simulink model "Classical_PTC_simo"  (R2016a)
settings: Solver=FixedStepAuto  StartTime=0.0  StopTime=3.8  FixedStep=1e-6  MaxStep=4e-6  RelTol=1e-6
values from neighbouring files (symbols this model uses):
  alpbet = [2/3, -1/3, -1/3; 0, sqrt(3)/3, -sqrt(3)/3 ]    [params_for_simo_Nisan21.m]
  kr = Lm/Lr    (= 0.98)    [params_for_simo_Nisan21.m]
  Lambda = 50    [params_for_simo_Nisan21.m]
  NTlimit = -3    [params_for_simo_Nisan21.m]
  OCLimit = 10    [params_for_simo_Nisan21.m]
  PhisRef = 0.3    [params_for_simo_Nisan21.m]
  PP = 1    [params_for_simo_Nisan21.m]
  PTlimit = 3    [params_for_simo_Nisan21.m]
  Req = Rs+kr*kr*Rr    (= 5.27724)    [params_for_simo_Nisan21.m]
  Rs = 2.3    [params_for_simo_Nisan21.m]
  taur = Lr/Rr    (= 0.0322580645161)    [params_for_simo_Nisan21.m]
  taus = Lstr/Req    (= 0.00112937823559)    [params_for_simo_Nisan21.m]
  Tmpc = T    (= 2.5e-05)    [params_for_simo_Nisan21.m]
undefined symbols (not defined in the file or in its folder): DiscIntNeverNeededParam
libraries: powerlib x7, simulink x2
settings Model: NumberOfSteps=30  Creator=pc  LastModifiedBy=silker
settings SolverCC: AlgebraicLoopSolver=LineSearch

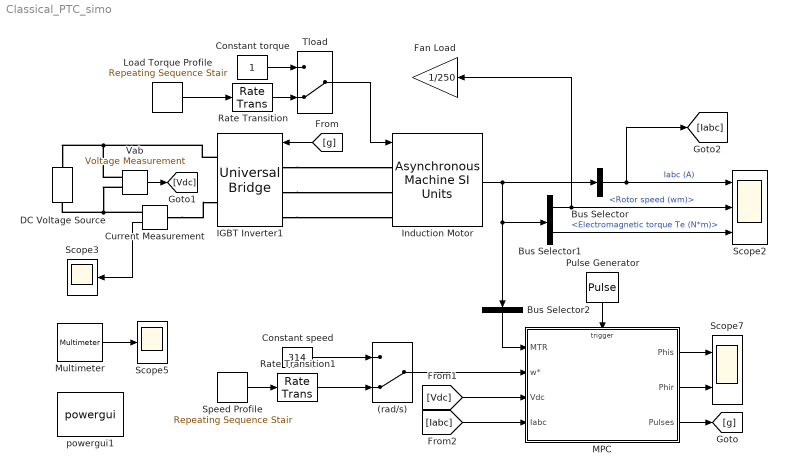
== system Classical_PTC_simo ==
  (rad/s) : ManualSwitch  CurrentSetting=0
  Bus Selector : BusSelector  OutputSignals=Stator measurements.Stator current is_a (A),Stator measurements.Stator current is_b (A),Stator measurements.Stator current is_c (A)  OutputAsBus=on
  Bus Selector1 : BusSelector  OutputSignals=Mechanical.Rotor speed (wm),Mechanical.Electromagnetic torque Te (N*m)
  Bus Selector2 : BusSelector  OutputSignals=Stator measurements.Stator flux phis_q (V s),Stator measurements.Stator flux phis_d (V s),Rotor measurements.Rotor flux phir_q (V s),Rotor measurements.Rotor flux phir_d (V s),Mechanical.Rotor speed (wm)  OutputAsBus=on
  Constant speed : Constant  Value=314
  Constant torque : Constant
  Current Measurement : powerlib/Measurements/Current Measurement  PhasorSimulation=off  OutputType=Complex  PSBequivalent=0
  DC Voltage Source : powerlib/Electrical Sources/DC Voltage Source  Amplitude=350  Measurements=None
  Fan Load : Gain  Gain=1/250
  IGBT Inverter1 : powerlib/Power Electronics/Universal Bridge  Arms=3  SnubberResistance=1e6  SnubberCapacitance=1e-9  Device=IGBT / Diodes  Ron=1e-3  Lon=0  ForwardVoltages="[  0.8  0.8  ]"  ForwardVoltage=.8  GTOparameters=[ 1e-6 , 1e-6 ]  IGBTparameters=[ 1e-6 , 2e-6 ]  Measurements=All voltages and currents  Measurements_2=None  converterType=Rectifier
  Induction Motor : powerlib/Machines/Asynchronous Machine SI Units  RotorType=Squirrel-cage  PresetModel=No  MechanicalLoad=Torque Tm  ShowDetailedParameters=on  ReferenceFrame=Stationary  Units=SI  MeasurementBus=off  NominalParameters=[ 1500, 380, 50 ]  Stator=[ 2.3 4e-3 ]  Rotor="[3.1  2e-3 ]"  Cage1=[ 0.022 0.226/377]  Cage2=[ 0.022 0.226/377]  Lm=98e-3  Mechanical="[0.003  0.0005 1 ]"  PolePairs=2  InitialConditions="[ 1, 0 ,  0 , 0 , 0 , 0 , 0 , 0 ]"  SimulateSaturation=off  Saturation=[0 0;0 0]  LoadFlowParameters=0  TsPowergui=0  TsBlock=-1  IterativeModel=Trapezoidal non iterative  IterativeDiscreteModel=Trapezoidal non iterative  Pmec=0
  Load Torque Profile : simulink/Sources/Repeating Sequence Stair  OutValues="[0.7 0.7 0.7 0.7 0.7 0.7 0.7 0.7 0.7 0.7 1.35 1.35 1.35 1.35 1.35 1.35 1.35 1.35 1.35  -0.3 -0.3 -0.3 -0.3 -0.3 -0.3 -0.3 -0.3 -0.3 -0.3 -1.35 -1.35 -1.35 -1.35 -1.35 -0.7 -0.7 -0.7 -0.7 ]"  tsamp=0.1  OutMin=[]  OutMax=[]  OutDataTypeStr=double  OutputDataTypeScalingMode=double  OutDataType=fixdt(0,8)  ConRadixGroup=Best Precision: Vector-wise  OutScaling=2^-12
  MPC : Subsystem  TreatAsAtomicUnit=on
  Multimeter : powerlib/Measurements/Multimeter  PhasorSimulation=off  OutputType=Complex  sel=11  L=16  Gain=1  yselected={'Isw1: IGBT Inverter1'};  PSBOutputType=1  PSBequivalent=0  AxesSetting=[0,0.1,-100,100]  Display=0  SavedBlockNames=-11
  Pulse Generator : DiscretePulseGenerator  PulseType=Time based  Period=Tmpc  PulseWidth=40
  Rate Transition : RateTransition  X0=0.7
  Rate Transition1 : RateTransition  X0=300
  Scope2 : Scope  NumInputPorts=3
  Scope3 : Scope
  Scope5 : Scope
  Scope7 : Scope  NumInputPorts=2
  Speed Profile : simulink/Sources/Repeating Sequence Stair  OutValues=[ 300 300 300 300 300 300 300 150 150 150 150 150 150 300 300 300 300 300 300 -300 -300 -300 -300 -300 -300 -300 -300 -300 -300 -300 -300 -150 -150 -150 -150 -150 -150 -150]  tsamp=0.1  OutMin=[]  OutMax=[]  OutDataTypeStr=double  OutputDataTypeScalingMode=double  OutDataType=fixdt(0,8)  ConRadixGroup=Best Precision: Vector-wise  OutScaling=2^-12
  Tload : ManualSwitch  CurrentSetting=0
  Vab : powerlib/Measurements/Voltage Measurement  Tag=PoWeRsYsTeMmEaSuReMeNt  PhasorSimulation=off  OutputType=Magnitude  PSBequivalent=0
  powergui1 : powerlib/powergui  Priority=1  SimulationMode=Discrete  SolverType=Tustin/Backward Euler (TBE)  SampleTime=1e-6  frequency=60  SPID=off  DisableSnubberDevices=off  DisableRonSwitches=off  DisableVfSwitches=off  SwTol=0  DisplayEquations=off  Interpol=off  ExternalGateDelay=off  methode=off  Ts=10  FunctionMessages=off  echomessages=off  HookPort=off  EnableUseOfTLC=off  x0status=blocks  frequencyindice=0  Pbase=100e6  ErrMax=1e-4  Iterations=50  UnitsV=kV  UnitsW=MW  buscounter=0  RestoreLinks=warning  ResistiveCurrentMeasurement=off  Frange=[0:2:500]  Ylog=off  Xlog=on  ShowGrid=off  save=off  variable=ZData  structure=classical_cur  ZoomFFT=off  StartTime=0.305  cycles=20  DisplayStyle=1  fundamental=33  FreqAxis=off  MaxFrequency=10000  frequencyindicesteady=1  RmsSteady=1  display=off
  wires:
  Pulse Generator/1 -> MPC/Trigger
  Load Torque Profile/1 -> Rate Transition/1
  Constant torque/1 -> Tload/1
  Induction Motor/1 -> Bus Selector/1, Bus Selector2/1, Bus Selector1/1
  Bus Selector2/1 -> MPC/1(MTR)
  MPC/3(Pulses) -> [g]
  [g] -> IGBT Inverter1/1
  Constant speed/1 -> (rad/s)/1
  Rate Transition1/1 -> (rad/s)/2
  Vab/1 -> [Vdc]
  [Vdc] -> MPC/3(Vdc)
  Rate Transition/1 -> Tload/2
  Current Measurement/1 -> Scope3/1
  (rad/s)/1 -> MPC/2(w*)
  Bus Selector1/1 -> Scope2/2, Fan Load/1  "<Rotor speed (wm)>"
  Bus Selector1/2 -> Scope2/3  "<Electromagnetic torque Te (N*m)>"
  [Iabc] -> MPC/4(Iabc)
  Bus Selector/1 -> Scope2/1, [Iabc]  "Iabc (A)"
  Multimeter/1 -> Scope5/1
  MPC/1(Phis) -> Scope7/1
  MPC/2(Phir) -> Scope7/2
  Speed Profile/1 -> Rate Transition1/1
  Tload/1 -> Induction Motor/1
  connections:
  Vab/LConn2 -- DC Voltage Source/LConn1 -- Current Measurement/RConn1
  IGBT Inverter1/RConn1 -- Vab/LConn1 -- DC Voltage Source/RConn1
  IGBT Inverter1/LConn1 -- Induction Motor/LConn1
  IGBT Inverter1/LConn2 -- Induction Motor/LConn2
  IGBT Inverter1/LConn3 -- Induction Motor/LConn3
  Current Measurement/LConn1 -- IGBT Inverter1/RConn2

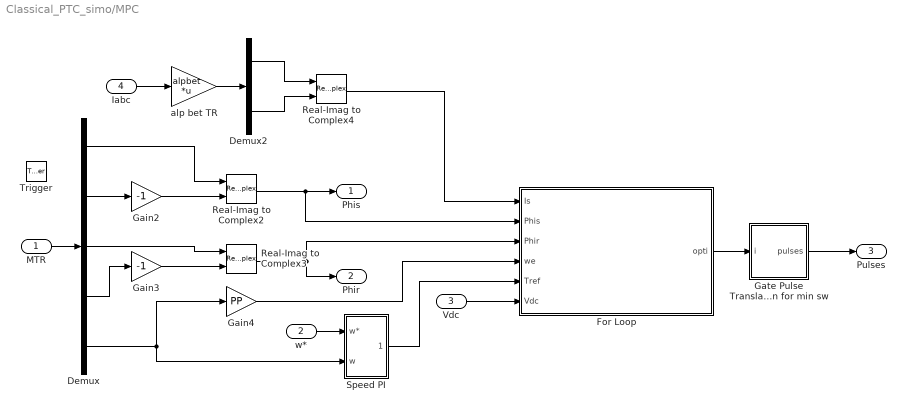
== system Classical_PTC_simo/MPC ==
  MTR : Inport
  w* : Inport  Port=2
  Vdc : Inport  Port=3
  Iabc : Inport  Port=4
  Trigger : TriggerPort  VariantControl=Variant
  Demux : Demux  Outputs=5
  Demux2 : Demux  Outputs=2
  For Loop : Subsystem  TreatAsAtomicUnit=on
  Gain2 : Gain  Gain=-1
  Gain3 : Gain  Gain=-1
  Gain4 : Gain  Gain=PP
  Gate Pulse Translation for min sw : Subsystem
  Real-Imag to Complex2 : RealImagToComplex
  Real-Imag to Complex3 : RealImagToComplex
  Real-Imag to Complex4 : RealImagToComplex
  Speed PI : Subsystem
  alp bet TR : Gain  Gain=alpbet  Multiplication=Matrix(K*u)
  Phis : Outport
  Phir : Outport  Port=2
  Pulses : Outport  Port=3
  wires:
  MTR/1 -> Demux/1
  Gain3/1 -> Real-Imag to Complex3/2
  Gain2/1 -> Real-Imag to Complex2/2
  Real-Imag to Complex2/1 -> For Loop/2(Phis), Phis/1
  Real-Imag to Complex3/1 -> For Loop/3(Phir), Phir/1
  w*/1 -> Speed PI/1(w*)
  Gain4/1 -> For Loop/4(we)
  Speed PI/1(Te*) -> For Loop/5(Tref)
  Vdc/1 -> For Loop/6(Vdc)
  Gate Pulse Translation for min sw/1(pulses) -> Pulses/1
  For Loop/1(opti) -> Gate Pulse Translation for min sw/1(i)
  Demux/1 -> Real-Imag to Complex2/1
  Demux/2 -> Gain2/1
  Demux/3 -> Real-Imag to Complex3/1
  Demux/4 -> Gain3/1
  Demux/5 -> Gain4/1, Speed PI/2(w)
  Iabc/1 -> alp bet TR/1
  Demux2/2 -> Real-Imag to Complex4/2
  Demux2/1 -> Real-Imag to Complex4/1
  alp bet TR/1 -> Demux2/1
  Real-Imag to Complex4/1 -> For Loop/1(Is)

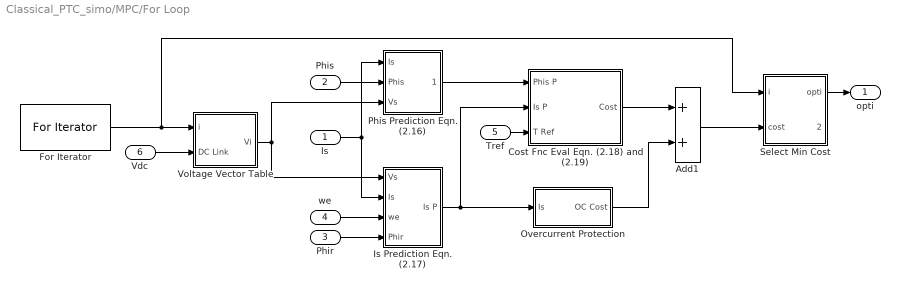
== system Classical_PTC_simo/MPC/For Loop ==
  Is : Inport
  Phis : Inport  Port=2
  Phir : Inport  Port=3
  we : Inport  Port=4
  Tref : Inport  Port=5
  Vdc : Inport  Port=6
  Add1 : Sum
  Cost Fnc Eval Eqn. (2.18) and (2.19) : Subsystem
  For Iterator : ForIterator  IterationLimit=7  IterationVariableDataType=double
  Is Prediction Eqn. (2.17) : Subsystem
  Overcurrent Protection : Subsystem
  Phis Prediction Eqn. (2.16) : Subsystem
  Select Min Cost : Subsystem
  Voltage Vector Table : Subsystem
  opti : Outport
  wires:
  Select Min Cost/1(opti) -> opti/1
  Voltage Vector Table/1(Vi) -> Phis Prediction Eqn. (2.16)/3(Vs), Is Prediction Eqn. (2.17)/1(Vs)
  Phis Prediction Eqn. (2.16)/1(Phis P) -> Cost Fnc Eval Eqn. (2.18) and (2.19)/1(Phis P)
  Is Prediction Eqn. (2.17)/1(Is P) -> Overcurrent Protection/1(Is), Cost Fnc Eval Eqn. (2.18) and (2.19)/2(Is P)
  Cost Fnc Eval Eqn. (2.18) and (2.19)/1(Cost) -> Add1/1
  Overcurrent Protection/1(OC Cost) -> Add1/2
  Is/1 -> Is Prediction Eqn. (2.17)/2(Is), Phis Prediction Eqn. (2.16)/1(Is)
  Phis/1 -> Phis Prediction Eqn. (2.16)/2(Phis)
  Phir/1 -> Is Prediction Eqn. (2.17)/4(Phir)
  we/1 -> Is Prediction Eqn. (2.17)/3(we)
  Vdc/1 -> Voltage Vector Table/2(DC Link)
  Tref/1 -> Cost Fnc Eval Eqn. (2.18) and (2.19)/3(T Ref)
  Add1/1 -> Select Min Cost/2(cost)
  For Iterator/1 -> Select Min Cost/1(i), Voltage Vector Table/1(i)

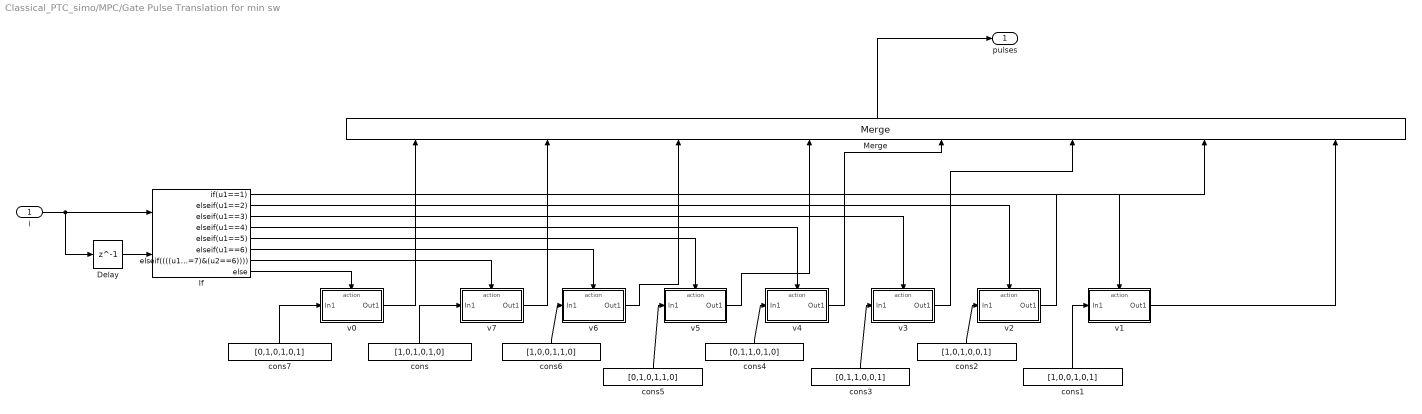
== system Classical_PTC_simo/MPC/Gate Pulse Translation for min sw ==
  i : Inport
  Delay : Delay  DelayLength=1  InitialCondition=0
  If : If  NumInputs=2  IfExpression=u1==1  ElseIfExpressions=u1==2, u1==3, u1==4, u1==5, u1==6,(((u1==7)&(u2==2)) | ((u1==7)&(u2==4)) | ((u1==7)&(u2==6)))
  Merge : Merge  Inputs=8
  cons : Constant  Value=[1,0,1,0,1,0]
  cons1 : Constant  Value=[1,0,0,1,0,1]
  cons2 : Constant  Value=[1,0,1,0,0,1]
  cons3 : Constant  Value=[0,1,1,0,0,1]
  cons4 : Constant  Value=[0,1,1,0,1,0]
  cons5 : Constant  Value=[0,1,0,1,1,0]
  cons6 : Constant  Value=[1,0,0,1,1,0]
  cons7 : Constant  Value=[0,1,0,1,0,1]
  v0 : Subsystem  TreatAsAtomicUnit=on
  v1 : Subsystem  TreatAsAtomicUnit=on
  v2 : Subsystem  TreatAsAtomicUnit=on
  v3 : Subsystem  TreatAsAtomicUnit=on
  v4 : Subsystem  TreatAsAtomicUnit=on
  v5 : Subsystem  TreatAsAtomicUnit=on
  v6 : Subsystem  TreatAsAtomicUnit=on
  v7 : Subsystem  TreatAsAtomicUnit=on
  pulses : Outport
  wires:
  i/1 -> Delay/1, If/1
  If/1 -> v1/Action
  Merge/1 -> pulses/1
  cons/1 -> v7/1(In1)
  If/3 -> v3/Action
  If/2 -> v2/Action
  If/4 -> v4/Action
  If/5 -> v5/Action
  If/7 -> v7/Action
  If/6 -> v6/Action
  cons1/1 -> v1/1(In1)
  cons2/1 -> v2/1(In1)
  cons3/1 -> v3/1(In1)
  cons4/1 -> v4/1(In1)
  cons5/1 -> v5/1(In1)
  cons6/1 -> v6/1(In1)
  Delay/1 -> If/2
  cons7/1 -> v0/1(In1)
  If/8 -> v0/Action
  v0/1(Out1) -> Merge/1
  v7/1(Out1) -> Merge/2
  v6/1(Out1) -> Merge/3
  v5/1(Out1) -> Merge/4
  v4/1(Out1) -> Merge/5
  v3/1(Out1) -> Merge/6
  v2/1(Out1) -> Merge/7
  v1/1(Out1) -> Merge/8

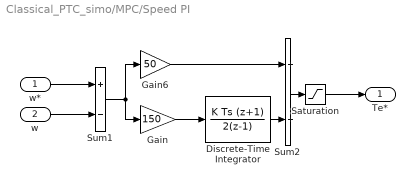
== system Classical_PTC_simo/MPC/Speed PI ==
  w* : Inport
  w : Inport  Port=2
  Discrete-Time Integrator : DiscreteIntegrator  IntegratorMethod=Integration: Trapezoidal  SampleTime=-1  LimitOutput=on  UpperSaturationLimit=90  LowerSaturationLimit=-90  ICPrevOutput=DiscIntNeverNeededParam  ICPrevScaledInput=DiscIntNeverNeededParam
  Gain : Gain  Gain=150  SaturateOnIntegerOverflow=on  OutDataTypeStr=Inherit: Same as input  ParamDataTypeStr=Inherit: Same as input
  Gain6 : Gain  Gain=50  SaturateOnIntegerOverflow=on  OutDataTypeStr=Inherit: Same as input  ParamDataTypeStr=Inherit: Same as input
  Saturation : Saturate  UpperLimit=PTlimit  LowerLimit=NTlimit
  Sum1 : Sum  Inputs=+-  SaturateOnIntegerOverflow=on  InputSameDT=on  OutDataTypeStr=Inherit: Same as first input
  Sum2 : Sum  SaturateOnIntegerOverflow=on  InputSameDT=on  OutDataTypeStr=Inherit: Same as first input
  Te* : Outport  InitialOutput=0
  wires:
  Gain/1 -> Discrete-Time Integrator/1
  Sum1/1 -> Gain/1, Gain6/1
  Gain6/1 -> Sum2/1
  Saturation/1 -> Te*/1
  w*/1 -> Sum1/1
  w/1 -> Sum1/2
  Discrete-Time Integrator/1 -> Sum2/2
  Sum2/1 -> Saturation/1

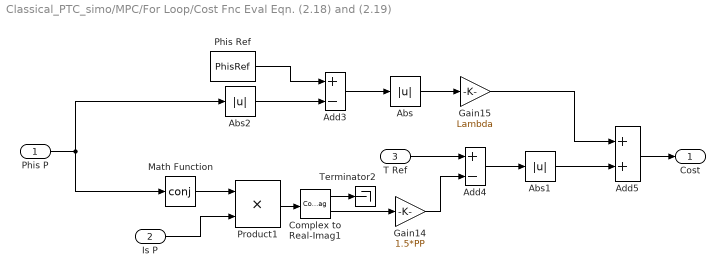
== system Classical_PTC_simo/MPC/For Loop/Cost Fnc Eval Eqn. (2.18) and (2.19) ==
  Phis P : Inport
  Is P : Inport  Port=2
  T Ref : Inport  Port=3
  Abs : Abs
  Abs1 : Abs
  Abs2 : Abs
  Add3 : Sum  Inputs=+-
  Add4 : Sum  Inputs=+-
  Add5 : Sum
  Complex to Real-Imag1 : ComplexToRealImag
  Gain14 : Gain  Gain=1.5*PP
  Gain15 : Gain  Gain=Lambda
  Math Function : Math  Operator=conj  SaturateOnIntegerOverflow=on
  Phis Ref : Constant  Value=PhisRef
  Product1 : Product
  Terminator2 : Terminator
  Cost : Outport
  wires:
  Phis P/1 -> Abs2/1, Math Function/1
  Complex to Real-Imag1/1 -> Terminator2/1
  Is P/1 -> Product1/2
  Product1/1 -> Complex to Real-Imag1/1
  Math Function/1 -> Product1/1
  Add3/1 -> Abs/1
  Gain14/1 -> Add4/2
  Phis Ref/1 -> Add3/1
  T Ref/1 -> Add4/1
  Abs1/1 -> Add5/2
  Add5/1 -> Cost/1
  Add4/1 -> Abs1/1
  Gain15/1 -> Add5/1
  Abs/1 -> Gain15/1
  Complex to Real-Imag1/2 -> Gain14/1
  Abs2/1 -> Add3/2

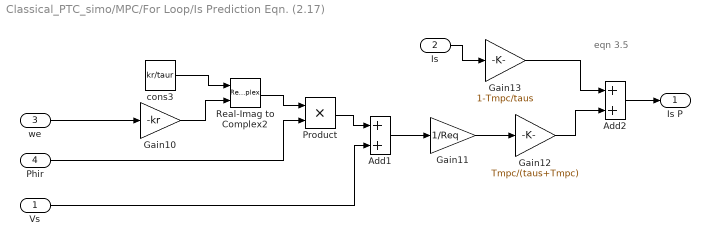
== system Classical_PTC_simo/MPC/For Loop/Is Prediction Eqn. (2.17) ==
  note: eqn 3.5
  Vs : Inport
  Is : Inport  Port=2
  we : Inport  Port=3
  Phir : Inport  Port=4
  Add1 : Sum
  Add2 : Sum
  Gain10 : Gain  Gain=-kr
  Gain11 : Gain  Gain=1/Req
  Gain12 : Gain  Gain=Tmpc/(taus+Tmpc)
  Gain13 : Gain  Gain=1-Tmpc/taus
  Product : Product
  Real-Imag to Complex2 : RealImagToComplex
  cons3 : Constant  Value=kr/taur
  Is P : Outport
  wires:
  Gain12/1 -> Add2/2
  Gain10/1 -> Real-Imag to Complex2/2
  Gain11/1 -> Gain12/1
  Product/1 -> Add1/1
  Phir/1 -> Product/2
  Gain13/1 -> Add2/1
  Vs/1 -> Add1/2
  cons3/1 -> Real-Imag to Complex2/1
  we/1 -> Gain10/1
  Real-Imag to Complex2/1 -> Product/1
  Add1/1 -> Gain11/1
  Add2/1 -> Is P/1
  Is/1 -> Gain13/1

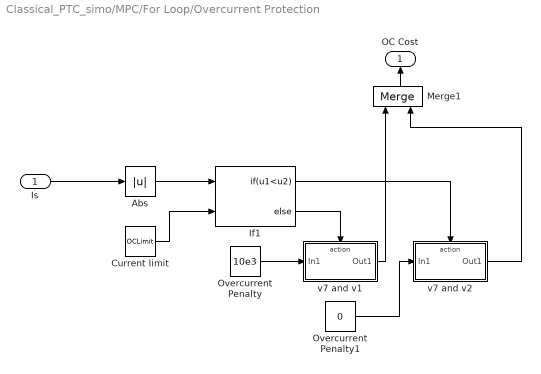
== system Classical_PTC_simo/MPC/For Loop/Overcurrent Protection ==
  Is : Inport
  Abs : Abs
  Current limit : Constant  Value=OCLimit
  If1 : If  NumInputs=2  IfExpression=u1<u2
  Merge1 : Merge
  Overcurrent Penalty : Constant  Value=10e3
  Overcurrent Penalty1 : Constant  Value=0
  v7 and v1 : Subsystem  TreatAsAtomicUnit=on
  v7 and v2 : Subsystem  TreatAsAtomicUnit=on
  OC Cost : Outport
  wires:
  Overcurrent Penalty/1 -> v7 and v1/1(In1)
  Merge1/1 -> OC Cost/1
  Abs/1 -> If1/1
  Overcurrent Penalty1/1 -> v7 and v2/1(In1)
  v7 and v2/1(Out1) -> Merge1/2
  v7 and v1/1(Out1) -> Merge1/1
  If1/1 -> v7 and v2/Action
  If1/2 -> v7 and v1/Action
  Is/1 -> Abs/1
  Current limit/1 -> If1/2

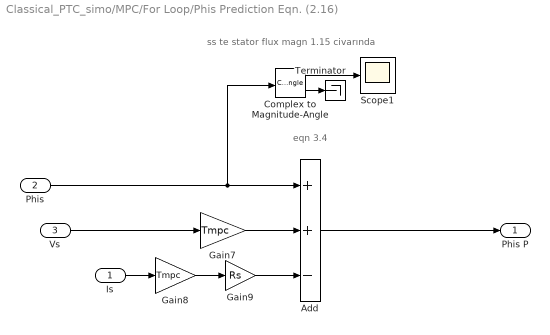
== system Classical_PTC_simo/MPC/For Loop/Phis Prediction Eqn. (2.16) ==
  note: ss te stator flux magn 1.15 civarında
  note: eqn 3.4
  Is : Inport
  Phis : Inport  Port=2
  Vs : Inport  Port=3
  Add : Sum  Inputs=++-
  Complex to Magnitude-Angle : ComplexToMagnitudeAngle
  Gain7 : Gain  Gain=Tmpc
  Gain8 : Gain  Gain=Tmpc
  Gain9 : Gain  Gain=Rs
  Scope1 : Scope
  Terminator : Terminator
  Phis P : Outport
  wires:
  Is/1 -> Gain8/1
  Complex to Magnitude-Angle/2 -> Terminator/1
  Vs/1 -> Gain7/1
  Gain9/1 -> Add/3
  Phis/1 -> Complex to Magnitude-Angle/1, Add/1
  Gain7/1 -> Add/2
  Gain8/1 -> Gain9/1
  Complex to Magnitude-Angle/1 -> Scope1/1
  Add/1 -> Phis P/1

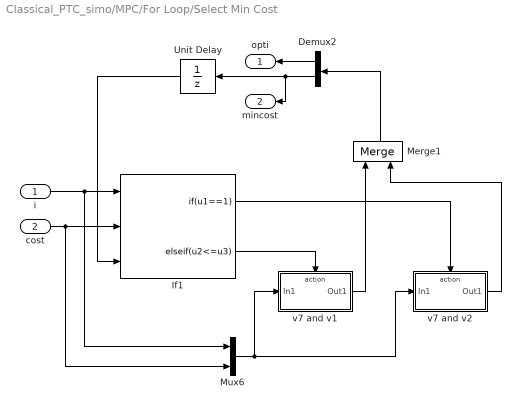
== system Classical_PTC_simo/MPC/For Loop/Select Min Cost ==
  i : Inport
  cost : Inport  Port=2
  Demux2 : Demux  Outputs=2
  If1 : If  NumInputs=3  IfExpression=u1==1  ElseIfExpressions=u2<=u3  ShowElse=off
  Merge1 : Merge
  Mux6 : Mux  Inputs=2
  Unit Delay : UnitDelay  SampleTime=-1
  v7 and v1 : Subsystem  TreatAsAtomicUnit=on
  v7 and v2 : Subsystem  TreatAsAtomicUnit=on
  opti : Outport
  mincost : Outport  Port=2
  wires:
  cost/1 -> Mux6/2, If1/2
  If1/1 -> v7 and v2/Action
  Unit Delay/1 -> If1/3
  i/1 -> Mux6/1, If1/1
  Mux6/1 -> v7 and v1/1(In1), v7 and v2/1(In1)
  Merge1/1 -> Demux2/1
  Demux2/2 -> mincost/1, Unit Delay/1
  If1/2 -> v7 and v1/Action
  v7 and v1/1(Out1) -> Merge1/1
  v7 and v2/1(Out1) -> Merge1/2
  Demux2/1 -> opti/1

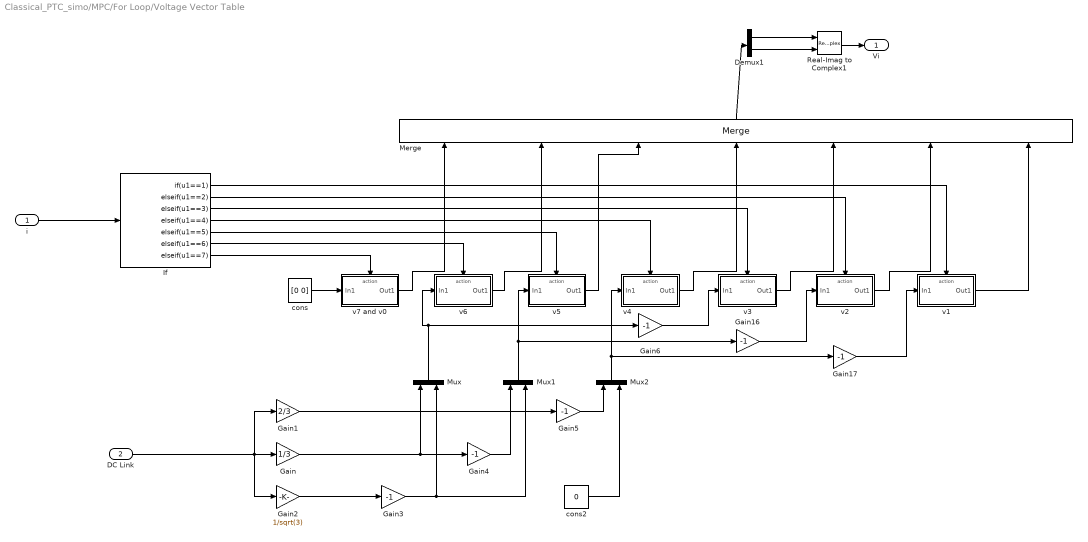
== system Classical_PTC_simo/MPC/For Loop/Voltage Vector Table ==
  i : Inport
  DC Link : Inport  Port=2
  Demux1 : Demux  Outputs=2
  Gain : Gain  Gain=1/3
  Gain1 : Gain  Gain=2/3
  Gain{3..6,16..17} (6 alike) : Gain  Gain=-1
  Gain2 : Gain  Gain=1/sqrt(3)
  If : If  IfExpression=u1==1  ElseIfExpressions=u1==2, u1==3, u1==4, u1==5, u1==6, u1==7  ShowElse=off
  Merge : Merge  Inputs=7
  Mux : Mux  Inputs=2
  Mux1 : Mux  Inputs=2
  Mux2 : Mux  Inputs=2
  Real-Imag to Complex1 : RealImagToComplex
  cons : Constant  Value=[0 0]
  cons2 : Constant  Value=0
  v1 : Subsystem  TreatAsAtomicUnit=on
  v2 : Subsystem  TreatAsAtomicUnit=on
  v3 : Subsystem  TreatAsAtomicUnit=on
  v4 : Subsystem  TreatAsAtomicUnit=on
  v5 : Subsystem  TreatAsAtomicUnit=on
  v6 : Subsystem  TreatAsAtomicUnit=on
  v7 and v0 : Subsystem  TreatAsAtomicUnit=on
  Vi : Outport
  wires:
  i/1 -> If/1
  Gain16/1 -> v2/1(In1)
  Gain6/1 -> v3/1(In1)
  Gain17/1 -> v1/1(In1)
  If/1 -> v1/Action
  Gain4/1 -> Mux1/1
  cons2/1 -> Mux2/2
  Merge/1 -> Demux1/1
  Gain1/1 -> Gain5/1
  cons/1 -> v7 and v0/1(In1)
  Gain2/1 -> Gain3/1
  Gain3/1 -> Mux1/2, Mux/2
  DC Link/1 -> Gain1/1, Gain/1, Gain2/1
  Mux2/1 -> Gain17/1, v4/1(In1)
  Mux1/1 -> Gain16/1, v5/1(In1)
  If/3 -> v3/Action
  Mux/1 -> Gain6/1, v6/1(In1)
  Demux1/2 -> Real-Imag to Complex1/2
  Gain5/1 -> Mux2/1
  If/2 -> v2/Action
  If/4 -> v4/Action
  If/5 -> v5/Action
  If/7 -> v7 and v0/Action
  Demux1/1 -> Real-Imag to Complex1/1
  If/6 -> v6/Action
  Gain/1 -> Gain4/1, Mux/1
  Real-Imag to Complex1/1 -> Vi/1
  v1/1(Out1) -> Merge/7
  v2/1(Out1) -> Merge/6
  v3/1(Out1) -> Merge/5
  v4/1(Out1) -> Merge/4
  v5/1(Out1) -> Merge/3
  v6/1(Out1) -> Merge/2
  v7 and v0/1(Out1) -> Merge/1

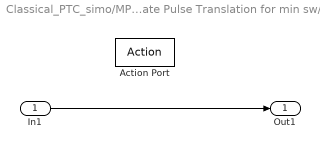
== system Classical_PTC_simo/MPC/Gate Pulse Translation for min sw/v0 ==
  In1 : Inport
  Action Port : ActionPort  ActionType=else
  Out1 : Outport
  wires:
  In1/1 -> Out1/1

== system Classical_PTC_simo/MPC/Gate Pulse Translation for min sw/v1 ==
  In1 : Inport
  Action Port : ActionPort  ActionType=then
  Out1 : Outport
  wires:
  In1/1 -> Out1/1

== system Classical_PTC_simo/MPC/Gate Pulse Translation for min sw/v2 ==
  In1 : Inport
  Action Port : ActionPort  ActionType=elseif
  Out1 : Outport
  wires:
  In1/1 -> Out1/1

== system Classical_PTC_simo/MPC/Gate Pulse Translation for min sw/v3 ==
  In1 : Inport
  Action Port : ActionPort  ActionType=elseif
  Out1 : Outport
  wires:
  In1/1 -> Out1/1

== system Classical_PTC_simo/MPC/Gate Pulse Translation for min sw/v4 ==
  In1 : Inport
  Action Port : ActionPort  ActionType=elseif
  Out1 : Outport
  wires:
  In1/1 -> Out1/1

== system Classical_PTC_simo/MPC/Gate Pulse Translation for min sw/v5 ==
  In1 : Inport
  Action Port : ActionPort  ActionType=elseif
  Out1 : Outport
  wires:
  In1/1 -> Out1/1

== system Classical_PTC_simo/MPC/Gate Pulse Translation for min sw/v6 ==
  In1 : Inport
  Action Port : ActionPort  ActionType=elseif
  Out1 : Outport
  wires:
  In1/1 -> Out1/1

== system Classical_PTC_simo/MPC/Gate Pulse Translation for min sw/v7 ==
  In1 : Inport
  Action Port : ActionPort  ActionType=elseif
  Out1 : Outport
  wires:
  In1/1 -> Out1/1

== system Classical_PTC_simo/MPC/For Loop/Overcurrent Protection/v7 and v1 ==
  In1 : Inport
  Action Port : ActionPort  ActionType=else
  Out1 : Outport
  wires:
  In1/1 -> Out1/1

== system Classical_PTC_simo/MPC/For Loop/Overcurrent Protection/v7 and v2 ==
  In1 : Inport
  Action Port : ActionPort  ActionType=then
  Out1 : Outport
  wires:
  In1/1 -> Out1/1

== system Classical_PTC_simo/MPC/For Loop/Select Min Cost/v7 and v1 ==
  In1 : Inport
  Action Port : ActionPort  ActionType=elseif
  Out1 : Outport
  wires:
  In1/1 -> Out1/1

== system Classical_PTC_simo/MPC/For Loop/Select Min Cost/v7 and v2 ==
  In1 : Inport
  Action Port : ActionPort  ActionType=then
  Out1 : Outport
  wires:
  In1/1 -> Out1/1

== system Classical_PTC_simo/MPC/For Loop/Voltage Vector Table/v1 ==
  In1 : Inport
  Action Port : ActionPort  ActionType=then
  Out1 : Outport
  wires:
  In1/1 -> Out1/1

== system Classical_PTC_simo/MPC/For Loop/Voltage Vector Table/v2 ==
  In1 : Inport
  Action Port : ActionPort  ActionType=elseif
  Out1 : Outport
  wires:
  In1/1 -> Out1/1

== system Classical_PTC_simo/MPC/For Loop/Voltage Vector Table/v3 ==
  In1 : Inport
  Action Port : ActionPort  ActionType=elseif
  Out1 : Outport
  wires:
  In1/1 -> Out1/1

== system Classical_PTC_simo/MPC/For Loop/Voltage Vector Table/v4 ==
  In1 : Inport
  Action Port : ActionPort  ActionType=elseif
  Out1 : Outport
  wires:
  In1/1 -> Out1/1

== system Classical_PTC_simo/MPC/For Loop/Voltage Vector Table/v5 ==
  In1 : Inport
  Action Port : ActionPort  ActionType=elseif
  Out1 : Outport
  wires:
  In1/1 -> Out1/1

== system Classical_PTC_simo/MPC/For Loop/Voltage Vector Table/v6 ==
  In1 : Inport
  Action Port : ActionPort  ActionType=elseif
  Out1 : Outport
  wires:
  In1/1 -> Out1/1

== system Classical_PTC_simo/MPC/For Loop/Voltage Vector Table/v7 and v0 ==
  In1 : Inport
  Action Port : ActionPort  ActionType=elseif
  Out1 : Outport
  wires:
  In1/1 -> Out1/1
